simulink model "RM3"  (R2018b)
settings: Solver=ode45  StartTime=0  StopTime=300  FixedStep=0.1  MaxStep=0.1  RelTol=1e-3  EnableMultiTasking=on
values from neighbouring files (symbols this model uses):
  waves = waveClass('regular')    [wecSimInputFile.m]    (also in wecSimInputFileold.m)
undefined symbols (not defined in the file or in its folder): body, constraint, pto, X, Y, Z
libraries: nesl_utility x9, sm_lib x5, WECSim_Lib x4
settings Model: Creator=mlawson  LastModifiedBy=David
settings SolverCC: ZeroCrossControl=DisableAll  AlgebraicLoopSolver=LineSearch  AutoInsertRateTranBlk=on
settings DataIOCC: SaveFormat=Array  SaveOutput=off  SaveTime=off
settings OptimizationCC: LifeSpan=inf  SimCompilerOptimization=on
settings DebuggingCC: UnderspecifiedInitializationDetection=Classic  MergeDetectMultiDrivingBlocksExec=none  SolverPrmCheckMsg=warning  AllowSymbolicDim=off  StateNameClashWarn=warning  SFUnexpectedBacktrackingDiag=warning  SFNoUnconditionalDefaultTransitionDiag=warning  SFExecutionAtInitializationDiag=none
settings HardwareCC: ProdBitPerPointer=32  ProdBitPerSizeT=32  ProdBitPerPtrDiffT=32  ProdLargestAtomicFloat=None  ProdIntDivRoundTo=Undefined  ProdEndianess=Unspecified  ProdWordSize=32  ProdHWDeviceType=32-bit Generic
settings ModelReferenceCC: PropagateSignalLabelsOutOfModel=off
settings SFSimCC: SimUseLocalCustomCode=off
settings RTWCC: RTWUseLocalCustomCode=off
settings CodeAppCC: StateflowObjectComments=on
settings GRTTargetCC: TargetLangStandard=C89/C90 (ANSI)  GeneratePreprocessorConditionals=Disable all
settings ConfigComp: CovMetricSettings=dw  CovHtmlReporting=on  CovSaveCumulativeToWorkspaceVar=on  CovSaveSingleToWorkspaceVar=on  CovExternalEMLEnable=off  CovSFcnEnable=off
settings SimscapeCC: SimscapeNormalizeSystem=off
settings ConfigurationSet: Description=SimMechanics 2G
settings ExplorerConfigSet: InternalSimMechanicsExplorerSettings="<ExplorerConfiguration><canonicalview>default</canonicalview><TilePanel><TileInfo><Tiles Columns=\"1\" Count=\"1\" Rows=\"1\"><Column Left=\"2\" Weight=\"1\"/><Column Left=\"1335\"/><Row Top=\"2\" Weight=\"1\"/><Row Top=\"911\"/><Tile Height=\"1\" Width=\"1\" X=\"0\" Y=\"0\"/></Tiles></TileInfo><SceneInfo><SceneViewer><BGColor><R>0.60000002384185791</R><G>0.60000002384185791</G><B>0.60000002384185791</B></BGColor><Camera><Position><X>365.37645888990272</X><Y>-369.82486814446582</Y><Z>359.64809521743916</Z></Position><Center><X>-6.7351450971904585</X><Y>2.2867358426280204</Y><Z>-12.463508769654169</Z></Center><Up><X>-0.40824829046386307</X><Y>0.40824829046386307</Y><Z>0.81649658092772615</Z></Up><Left>-57.820127362122818</Left><Right>57.820127362122818</Right><Bottom>-38.308817187253304</Bottom><Top>38.308817187253304</Top></Camera></SceneViewer></SceneInfo></TilePanel></ExplorerConfiguration>"

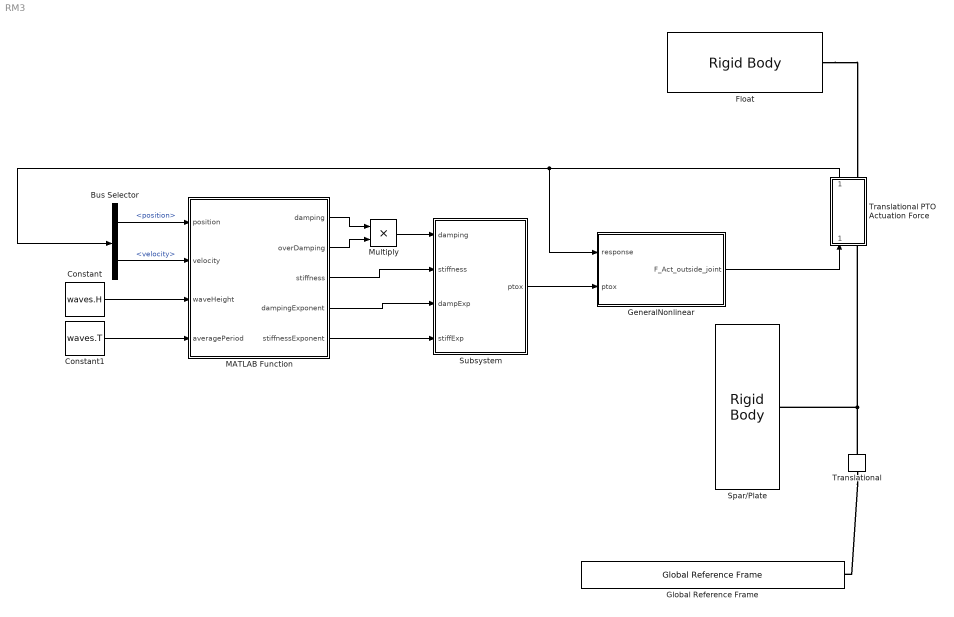
== system RM3 ==
  Bus Selector : BusSelector  OutputSignals=position,velocity
  Constant : Constant  Value=waves.H
  Constant1 : Constant  Value=waves.T
  Float : WECSim_Lib/Body Elements/Rigid Body  body=body(1)
      settings: AttributesFormatString=%<body>  SourceProductName=WEC-Sim
  GeneralNonlinear : Subsystem
  Global Reference Frame : WECSim_Lib/Frames/Global Reference Frame  waves=waves  simu=simu
      settings: SourceProductName=WEC-Sim
  MATLAB Function : MATLAB Function  TreatAsAtomicUnit=on
  Multiply : Product
  Spar/Plate : WECSim_Lib/Body Elements/Rigid Body  body=body(2)
      settings: AttributesFormatString=%<body>  SourceProductName=WEC-Sim
  Subsystem : Subsystem
  Translational : WECSim_Lib/Constraints/Translational  constraint=constraint(1)
      settings: AttributesFormatString=%<constraint>  SourceProductName=WEC-Sim
  Translational PTO Actuation Force : Subsystem  AncestorBlock=WECSim_Lib/PTOs/Translational PTO Actuation Force  mask(PTO){pto=pto(1)}
      mask prompts: pto "PTO Name:"
      mask help:
      | Constraints the follower to translational motion relative to the base, in
      | the PTO's Z-direction and adds PTO stiffness and damping. Also applies a
      | user-defined force and outputs extension, velocity, and acceleration.
      |
      |
      | The variable name input below must be 'pto(i)' where i=1,2,...
      | pto(i) must be defined in the input file with the following fields:
      |
      |     .name (required)
      |             String.
      |             PTO name. Must comply with Matlab's variable naming rules.
      |     .loc (optional)
      |             3x1 vector [x y z] in meters.
      |             PTO location. Default = [0 0 0]
      |     .k (optional)
      |             Float.
      |             PTO linear spring stiffness. Default = 0
      |     .c (optional)
      |             Float.
      |             PTO linear damping coefficient. Default = 0
      |     .orientation.z (optional)
      |             3x1 vector [x y z].
      |             Direction of the PTO's Z-coordinate. Default = [0 0 1]
      |     .orientation.y (optional)
      |             3x1 vector [x y z].
      |             Direction of the PTO's Y-coordinate. Default = [0 1 0]
      mask init:
      | if exist('pto','var')
      |     h=[gcb '/output'];
      |     responseName=['pto' num2str(pto.ptoNum) '_out'];
      |     set_param(h,'VariableName',responseName);
      | end
      | 
      | pto.checkLoc('W');
      settings: AttributesFormatString=%<pto>
      mask Help:
      | Constraints the follower to translational motion relative to the base, in
      | the PTO's Z-direction and adds PTO stiffness and damping. Also applies a
      | user-defined force and outputs extension, velocity, and acceleration.
      | 
      | 
      | The variable name input below must be 'pto(i)' where i=1,2,...
      | pto(i) must be defined in the input file with the following fields:
      | 
      |     .name (required)
      |             String.
      |             PTO name. Must comply with Matlab's variable naming rules.
      |     .loc (optional)
      |             3x1 vector [x y z] in meters.
      |             PTO location. Default = [0 0 0]
      |     .k (optional)
      |             Float.
      |             PTO linear spring stiffness. Default = 0
      |     .c (optional)
      |             Float.
      |             PTO linear damping coefficient. Default = 0
      |     .orientation.z (optional)
      |             3x1 vector [x y z].
      |             Direction of the PTO's Z-coordinate. Default = [0 0 1]
      |     .orientation.y (optional)
      |             3x1 vector [x y z].
      |             Direction of the PTO's Y-coordinate. Default = [0 1 0]
  wires:
  Translational PTO Actuation Force/1(Response) -> Bus Selector/1, GeneralNonlinear/1(response)
  GeneralNonlinear/1(F_Act_outside_joint) -> Translational PTO Actuation Force/1(Force)
  Subsystem/1(ptox) -> GeneralNonlinear/2(ptox)
  Bus Selector/1 -> MATLAB Function/1(position)  "<position>"
  Bus Selector/2 -> MATLAB Function/2(velocity)  "<velocity>"
  Constant/1 -> MATLAB Function/3(waveHeight)
  Constant1/1 -> MATLAB Function/4(averagePeriod)
  MATLAB Function/1(damping) -> Multiply/1
  MATLAB Function/2(overDamping) -> Multiply/2
  MATLAB Function/4(dampingExponent) -> Subsystem/3(dampExp)
  MATLAB Function/5(stiffnessExponent) -> Subsystem/4(stiffExp)
  Multiply/1 -> Subsystem/1(damping)
  MATLAB Function/3(stiffness) -> Subsystem/2(stiffness)
  connections:
  Translational/LConn1 -- Global Reference Frame/RConn1
  Translational/RConn1 -- Translational PTO Actuation Force/LConn1 -- Spar/Plate/RConn1
  Float/RConn1 -- Translational PTO Actuation Force/RConn1

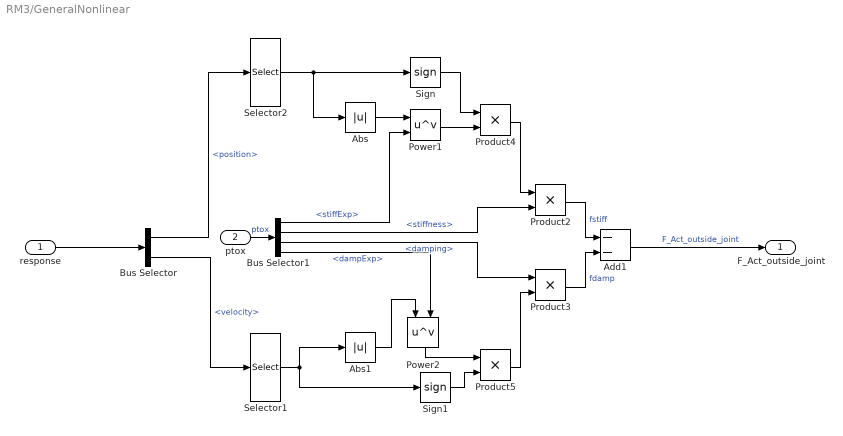
== system RM3/GeneralNonlinear ==
  response : Inport
  ptox : Inport  Port=2
  Abs : Abs
  Abs1 : Abs
  Add1 : Sum  Inputs=--
  Bus Selector : BusSelector  OutputSignals=position,velocity
  Bus Selector1 : BusSelector  OutputSignals=stiffExp,stiffness,damping,dampExp
  Power1 : Math  Operator=pow  SaturateOnIntegerOverflow=on
  Power2 : Math  Operator=pow  SaturateOnIntegerOverflow=on
  Product2 : Product  Inputs=**
  Product3 : Product  Inputs=**
  Product4 : Product
  Product5 : Product
  Selector1 : Selector  InputPortWidth=6  IndexOptions=Index vector (dialog)  Indices=3  OutputSizes=1
  Selector2 : Selector  InputPortWidth=6  IndexOptions=Index vector (dialog)  Indices=3  OutputSizes=1
  Sign : Signum
  Sign1 : Signum
  F_Act_outside_joint : Outport
  wires:
  Power2/1 -> Product5/1
  Product5/1 -> Product3/2
  Sign/1 -> Product4/1
  Bus Selector1/3 -> Product3/1  "<damping>"
  Product2/1 -> Add1/1  "fstiff"
  response/1 -> Bus Selector/1
  Bus Selector1/1 -> Power1/2  "<stiffExp>"
  Bus Selector/2 -> Selector1/1  "<velocity>"
  Selector2/1 -> Sign/1, Abs/1
  Product4/1 -> Product2/1
  Add1/1 -> F_Act_outside_joint/1  "F_Act_outside_joint"
  Abs1/1 -> Power2/1
  Product3/1 -> Add1/2  "fdamp"
  Sign1/1 -> Product5/2
  Bus Selector1/2 -> Product2/2  "<stiffness>"
  Selector1/1 -> Abs1/1, Sign1/1
  Power1/1 -> Product4/2
  Bus Selector/1 -> Selector2/1  "<position>"
  Abs/1 -> Power1/1
  ptox/1 -> Bus Selector1/1  "ptox"
  Bus Selector1/4 -> Power2/2  "<dampExp>"

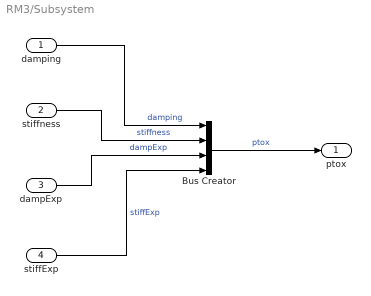
== system RM3/Subsystem ==
  damping : Inport
  stiffness : Inport  Port=2
  dampExp : Inport  Port=3
  stiffExp : Inport  Port=4
  Bus Creator : BusCreator  Inputs=4
  ptox : Outport
  wires:
  stiffness/1 -> Bus Creator/2  "stiffness"
  stiffExp/1 -> Bus Creator/4  "stiffExp"
  Bus Creator/1 -> ptox/1  "ptox"
  damping/1 -> Bus Creator/1  "damping"
  dampExp/1 -> Bus Creator/3  "dampExp"

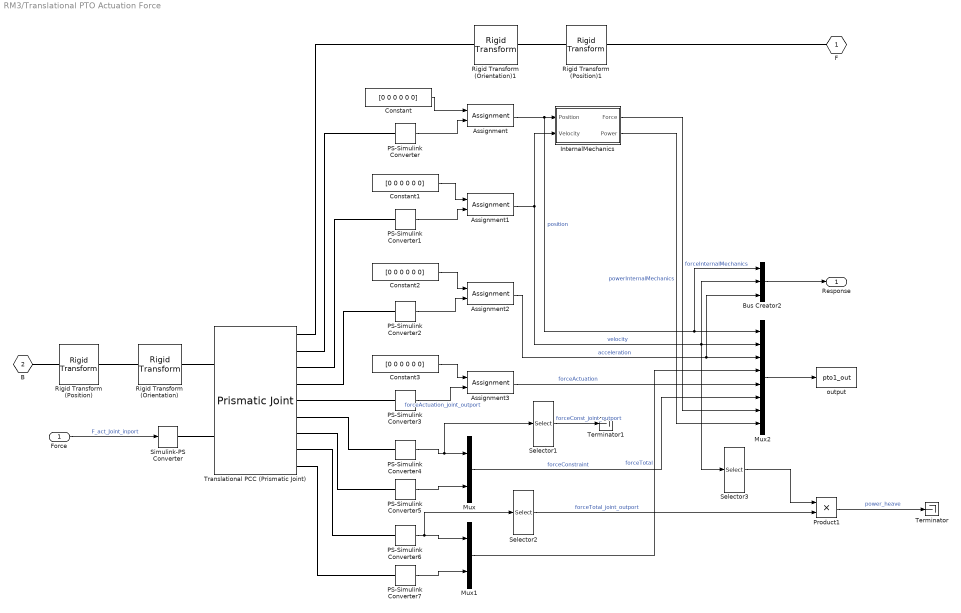
== system RM3/Translational PTO Actuation Force ==
  Force : Inport
  Assignment{,1..3} (4 alike) : Assignment  IndexOptions=Index vector (dialog)  Indices=3  OutputSizes=1
  Bus Creator2 : BusCreator  Inputs=3
  Constant{,1..3} (4 alike) : Constant  Value=[0 0 0 0 0 0]
  InternalMechanics : Subsystem
  Mux : Mux  Inputs=2
  Mux1 : Mux  Inputs=2
  Mux2 : Mux  Inputs=8
  PS-Simulink Converter{,1..7} (8 alike) : nesl_utility/PS-Simulink Converter  PhysicalDomain=network_engine_domain  SubClassName=ps_output  LeftPortType=input  RightPortType=output  PseudoPeriodic=off  Frequencies=[]  Unit=1  AffineConversion=off
  Product1 : Product
  Rigid Transform (Position) : sm_lib/Frames and Transforms/Rigid Transform  TranslationMethod=Cartesian  TranslationStandardOffset=0  TranslationLengthUnit=m  TranslationStandardAxis=+Z  TranslationCartesianOffset=pto.initDisp.initLinDisp + pto.loc  TranslationROffset=0  TranslationROffsetUnits=m  TranslationZOffset=0  TranslationZOffsetUnits=m  TranslationThetaOffset=0  TranslationThetaOffsetUnits=deg  RotationMethod=None  RotationAngleUnits=rad  RotationStandardAxis=+Y  RotationAngle=0  RotationArbitraryAxis=[0 1 0]  FollAlignAxisA=+X  BaseAlignAxisA=+Y  FollAlignAxisB=+Y  BaseAlignAxisB=+Z  RotationSequenceAxes=FollowerAxes  RotationSequence=XYX  RotationSequenceAngles=[0 0 0]  RotationSequenceAnglesUnits=deg  RotationMatrix=[1 0 0; 0 1 0; 0 0 1]
  Rigid Transform (Position)1 : sm_lib/Frames and Transforms/Rigid Transform  TranslationMethod=Cartesian  TranslationStandardOffset=0  TranslationLengthUnit=m  TranslationStandardAxis=+Z  TranslationCartesianOffset=pto.initDisp.initLinDisp + pto.loc  TranslationROffset=0  TranslationROffsetUnits=m  TranslationZOffset=0  TranslationZOffsetUnits=m  TranslationThetaOffset=0  TranslationThetaOffsetUnits=deg  RotationMethod=None  RotationAngleUnits=rad  RotationStandardAxis=+Y  RotationAngle=0  RotationArbitraryAxis=[0 1 0]  FollAlignAxisA=+X  BaseAlignAxisA=+Y  FollAlignAxisB=+Y  BaseAlignAxisB=+Z  RotationSequenceAxes=FollowerAxes  RotationSequence=XYX  RotationSequenceAngles=[0 0 0]  RotationSequenceAnglesUnits=deg  RotationMatrix=[1 0 0; 0 1 0; 0 0 1]
  Rigid Transform (Orientation) : sm_lib/Frames and Transforms/Rigid Transform  TranslationMethod=None  TranslationStandardOffset=0  TranslationLengthUnit=m  TranslationStandardAxis=+Z  TranslationCartesianOffset=0  TranslationROffset=0  TranslationROffsetUnits=m  TranslationZOffset=0  TranslationZOffsetUnits=m  TranslationThetaOffset=0  TranslationThetaOffsetUnits=deg  RotationMethod=RotationMatrix  RotationAngleUnits=rad  RotationStandardAxis=+Y  RotationAngle=0  RotationArbitraryAxis=[0 1 0]  FollAlignAxisA=+X  BaseAlignAxisA=+Y  FollAlignAxisB=+Y  BaseAlignAxisB=+Z  RotationSequenceAxes=FollowerAxes  RotationSequence=XYX  RotationSequenceAngles=[0 0 0]  RotationSequenceAnglesUnits=deg  RotationMatrix=pto.orientation.rotationMatrix
  Rigid Transform (Orientation)1 : sm_lib/Frames and Transforms/Rigid Transform  TranslationMethod=None  TranslationStandardOffset=0  TranslationLengthUnit=m  TranslationStandardAxis=+Z  TranslationCartesianOffset=0  TranslationROffset=0  TranslationROffsetUnits=m  TranslationZOffset=0  TranslationZOffsetUnits=m  TranslationThetaOffset=0  TranslationThetaOffsetUnits=deg  RotationMethod=RotationMatrix  RotationAngleUnits=rad  RotationStandardAxis=+Y  RotationAngle=0  RotationArbitraryAxis=[0 1 0]  FollAlignAxisA=+X  BaseAlignAxisA=+Y  FollAlignAxisB=+Y  BaseAlignAxisB=+Z  RotationSequenceAxes=FollowerAxes  RotationSequence=XYX  RotationSequenceAngles=[0 0 0]  RotationSequenceAnglesUnits=deg  RotationMatrix=pto.orientation.rotationMatrix
  Selector1 : Selector  InputPortWidth=3  IndexOptions=Index vector (dialog)  Indices=3  OutputSizes=1
  Selector2 : Selector  InputPortWidth=3  IndexOptions=Index vector (dialog)  Indices=3  OutputSizes=1
  Selector3 : Selector  InputPortWidth=6  IndexOptions=Index vector (dialog)  Indices=3  OutputSizes=1
  Simulink-PS Converter : nesl_utility/Simulink-PS Converter  PhysicalDomain=network_engine_domain  SubClassName=ps_input  LeftPortType=input  RightPortType=output  PseudoPeriodic=off  Frequencies=[]  NoiseDistribution=none  NoiseParameters=[]  Unit=1  AffineConversion=off  FilteringAndDerivatives=zero  SimscapeFilterOrder=1  InputFilterTimeConstant=0.001  UdotUserProvided=1
  Terminator : Terminator
  Terminator1 : Terminator
  Translational PCC (Prismatic Joint) : sm_lib/Joints/Prismatic Joint  SenseConstraintForce=on  SenseConstraintForceX=off  SenseConstraintForceY=off  SenseConstraintForceZ=off  SenseConstraintTorque=on  SenseConstraintTorqueX=off  SenseConstraintTorqueY=off  SenseConstraintTorqueZ=off  SenseTotalForce=on  SenseTotalForceX=off  SenseTotalForceY=off  SenseTotalForceZ=off  SenseTotalTorque=on  SenseTotalTorqueX=off  SenseTotalTorqueY=off  SenseTotalTorqueZ=off  CompositeWrenchDir=BaseOnFollower  CompositeWrenchFrame=BaseFrame  EquilibriumPosition=0  EquilibriumPositionUnits=m  SpringStiffness=pto.k  SpringStiffnessUnits=N/m  DampingCoefficient=pto.c  DampingCoefficientUnits=N/(m/s)  TorqueActuationMode=InputTorque  MotionActuationMode=ComputedMotion  SensePosition=on  SenseVelocity=on  SenseAcceleration=on  SenseTorqueForce=on  PositionTargetSpecify=off  PositionTargetPriority=High  PositionTargetValue=0  PositionTargetValueUnits=m  VelocityTargetSpecify=off  VelocityTargetPriority=High  VelocityTargetValue=0  VelocityTargetValueUnits=m/s
  output : ToWorkspace  VariableName=pto1_out  SaveFormat=Structure With Time  SampleTime=-1
      settings: Decimation=round(simu.dtOut/simu.dt,0)
  F : PMIOPort  Side=Right
  B : PMIOPort  Port=2  Side=Left
  Response : Outport
  wires:
  Bus Creator2/1 -> Response/1
  Assignment/1 -> Mux2/1, Bus Creator2/1, InternalMechanics/1(Position)  "position"
  Assignment1/1 -> Selector3/1, Bus Creator2/2, Mux2/2, InternalMechanics/2(Velocity)  "velocity"
  Assignment2/1 -> Mux2/3, Bus Creator2/3  "acceleration"
  Force/1 -> Simulink-PS Converter/1  "F_act_Joint_inport"
  Mux2/1 -> output/1
  Mux/1 -> Mux2/6  "forceConstraint"
  Mux1/1 -> Mux2/4  "forceTotal"
  PS-Simulink Converter5/1 -> Mux/2
  PS-Simulink Converter6/1 -> Selector2/1, Mux1/1
  PS-Simulink Converter7/1 -> Mux1/2
  Assignment3/1 -> Mux2/5  "forceActuation"
  Constant/1 -> Assignment/1
  PS-Simulink Converter/1 -> Assignment/2
  Constant1/1 -> Assignment1/1
  PS-Simulink Converter1/1 -> Assignment1/2
  Constant2/1 -> Assignment2/1
  PS-Simulink Converter2/1 -> Assignment2/2
  InternalMechanics/1(Force) -> Mux2/7  "forceInternalMechanics"
  InternalMechanics/2(Power) -> Mux2/8  "powerInternalMechanics"
  Constant3/1 -> Assignment3/1
  PS-Simulink Converter3/1 -> Assignment3/2  "forceActuation_joint_outport"
  Selector2/1 -> Product1/2  "forceTotal_joint_outport"
  PS-Simulink Converter4/1 -> Selector1/1, Mux/1
  Selector1/1 -> Terminator1/1  "forceConst_joint_outport"
  Product1/1 -> Terminator/1  "power_heave"
  Selector3/1 -> Product1/1
  connections:
  Rigid Transform (Position)/RConn1 -- Rigid Transform (Orientation)/LConn1
  Rigid Transform (Position)1/RConn1 -- Rigid Transform (Orientation)1/LConn1
  Simulink-PS Converter/RConn1 -- Translational PCC (Prismatic Joint)/LConn2
  Rigid Transform (Orientation)/RConn1 -- Translational PCC (Prismatic Joint)/LConn1
  Rigid Transform (Position)/LConn1 -- B/RConn1
  Translational PCC (Prismatic Joint)/RConn5 -- PS-Simulink Converter3/LConn1
  Translational PCC (Prismatic Joint)/RConn9 -- PS-Simulink Converter7/LConn1
  Rigid Transform (Orientation)1/RConn1 -- Translational PCC (Prismatic Joint)/RConn1
  Translational PCC (Prismatic Joint)/RConn4 -- PS-Simulink Converter2/LConn1
  Translational PCC (Prismatic Joint)/RConn7 -- PS-Simulink Converter5/LConn1
  Translational PCC (Prismatic Joint)/RConn3 -- PS-Simulink Converter1/LConn1
  Rigid Transform (Position)1/LConn1 -- F/RConn1
  Translational PCC (Prismatic Joint)/RConn8 -- PS-Simulink Converter6/LConn1
  Translational PCC (Prismatic Joint)/RConn2 -- PS-Simulink Converter/LConn1
  Translational PCC (Prismatic Joint)/RConn6 -- PS-Simulink Converter4/LConn1

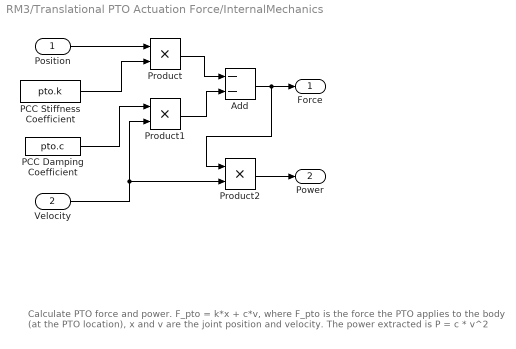
== system RM3/Translational PTO Actuation Force/InternalMechanics ==
  note: Calculate PTO force and power.
      |
      | F_pto  = k*x + c*v,
      | where F_pto is the force the PTO applies to the body (at the PTO location), x and v are the joint position and velocity.
      |
      | The power extracted is
      | P = c * v^2
  Position : Inport
  Velocity : Inport  Port=2
  Add : Sum  Inputs=--
  PCC Damping Coefficient : Constant  Value=pto.c
  PCC Stiffness Coefficient : Constant  Value=pto.k
  Product : Product  Inputs=**
  Product1 : Product  Inputs=**
  Product2 : Product  Inputs=**
  Force : Outport
  Power : Outport  Port=2
  wires:
  PCC Damping Coefficient/1 -> Product1/1
  Product2/1 -> Power/1
  PCC Stiffness Coefficient/1 -> Product/2
  Position/1 -> Product/1
  Add/1 -> Product2/1, Force/1
  Velocity/1 -> Product1/2, Product2/2
  Product/1 -> Add/1
  Product1/1 -> Add/2

== matlab function RM3/MATLAB Function ==
  data: position input; velocity input; waveHeight input; damping output; overDamping output; averagePeriod input; stiffness output; dampingExponent output; stiffnessExponent output
function [damping, overDamping, stiffness, dampingExponent, stiffnessExponent] =...
    fuzzyLogicController(position, velocity, waveHeight, averagePeriod)


start = tic;
verbose = 1;


%%%%%%%%%%%%%%%%%%%%%%%%%%%%%%%%%%%%%%%
%% Define input membership functions %%
%%%%%%%%%%%%%%%%%%%%%%%%%%%%%%%%%%%%%%%

%%% Waveheight Input %%%

    % Low waveheight open trap MF
    fS.inputs.waveHeight.MFs.low.type = 'down step';
    fS.inputs.waveHeight.MFs.low.begin = 0.41;
    fS.inputs.waveHeight.MFs.low.finish = 1.40;

    % Medium Low (Q1) waveheight triangular MF
    fS.inputs.waveHeight.MFs.medLow.type = 'triangle';
    fS.inputs.waveHeight.MFs.medLow.begin = 0.41;
    fS.inputs.waveHeight.MFs.medLow.peak = 1.40;
    fS.inputs.waveHeight.MFs.medLow.finish = 1.88;

    % Medium (median) waveheight triangular MF
    fS.inputs.waveHeight.MFs.med.type = 'triangle';
    fS.inputs.waveHeight.MFs.med.begin = 1.40;
    fS.inputs.waveHeight.MFs.med.peak = 1.88;
    fS.inputs.waveHeight.MFs.med.finish = 2.65;

    % Medium High (Q3) waveheight triangular MF
    fS.inputs.waveHeight.MFs.medHigh.type = 'triangle';
    fS.inputs.waveHeight.MFs.medHigh.begin = 1.88;
    fS.inputs.waveHeight.MFs.medHigh.peak = 2.65;
    fS.inputs.waveHeight.MFs.medHigh.finish = 10.43;

    % High waveheight open trap MF
    fS.inputs.waveHeight.MFs.high.type = 'step';
    fS.inputs.waveHeight.MFs.high.begin = 2.65;
    fS.inputs.waveHeight.MFs.high.finish = 10.43; 

%%% Average Wave Period Input %%%

    % Low period open trap MF
    fS.inputs.avgPeriod.MFs.short.type = 'down step';
    fS.inputs.avgPeriod.MFs.short.begin = 3.52;
    fS.inputs.avgPeriod.MFs.short.finish = 5.94;

    % Medium Low (Q1) period triangular MF
    fS.inputs.avgPeriod.MFs.midShort.type = 'triangle';
    fS.inputs.avgPeriod.MFs.midShort.begin = 3.52;
    fS.inputs.avgPeriod.MFs.midShort.peak = 5.94;
    fS.inputs.avgPeriod.MFs.midShort.finish = 6.81;

    % Medium (median) period triangular MF
    fS.inputs.avgPeriod.MFs.mid.type = 'triangle';
    fS.inputs.avgPeriod.MFs.mid.begin = 5.94;
    fS.inputs.avgPeriod.MFs.mid.peak = 6.81;
    fS.inputs.avgPeriod.MFs.mid.finish = 7.89;

    % Medium High (Q3) period triangular MF
    fS.inputs.avgPeriod.MFs.midLong.type = 'triangle';
    fS.inputs.avgPeriod.MFs.midLong.begin = 6.81;
    fS.inputs.avgPeriod.MFs.midLong.peak = 7.89;
    fS.inputs.avgPeriod.MFs.midLong.finish = 12.97;

    % High period open trap MF
    fS.inputs.avgPeriod.MFs.long.type = 'step';
    fS.inputs.avgPeriod.MFs.long.begin = 7.89;
    fS.inputs.avgPeriod.MFs.long.finish = 12.97;

%%% Velocity Input %%%

    % Too fast Negative Velocity Limit
    fS.inputs.velocity.MFs.fastNeg.type = 'down step';
    fS.inputs.velocity.MFs.fastNeg.begin = -1;
    fS.inputs.velocity.MFs.fastNeg.finish = 0;
    
    % In spec speeds
    fS.inputs.velocity.MFs.slow.type = 'triangle';
    fS.inputs.velocity.MFs.slow.begin = -1;
    fS.inputs.velocity.MFs.slow.peak = 0;
    fS.inputs.velocity.MFs.slow.finish = 1;
    
    % Too Fast Positive Velocity
    fS.inputs.velocity.MFs.fastPos.type = 'step';
    fS.inputs.velocity.MFs.fastPos.begin = 0;
    fS.inputs.velocity.MFs.fastPos.finish = 1;

%%% Position Input %%%

    % Too Negative Position Limit
    fS.inputs.position.MFs.low.type = 'down step';
    fS.inputs.position.MFs.low.begin = -1;
    fS.inputs.position.MFs.low.finish = -0.75;
    
    % In spec speeds
    fS.inputs.position.MFs.middle.type = 'trap';
    fS.inputs.position.MFs.middle.begin = -1;
    fS.inputs.position.MFs.middle.asc = -0.75;
    fS.inputs.position.MFs.middle.dec = 0.75;
    fS.inputs.position.MFs.middle.finish = 1;
    
    % Too Positive Position
    fS.inputs.position.MFs.high.type = 'step';
    fS.inputs.position.MFs.high.begin = 0.75;
    fS.inputs.position.MFs.high.finish = 1;

%%%%%%%%%%%%%%%%%%
%% Define Rules %%
%%%%%%%%%%%%%%%%%%
% Define Rules for outputs, Define Fuzzy Operators, (for speed and position, 
% any rule with multiple inputs), define each rule's implication method,
% define aggregation method for determining outputs for all rules 





%%%%%%%%%%%%%%%%%%
%% Fuzzify Inputs %%
%%%%%%%%%%%%%%%%%%
fS.inputs.waveHeight.MFs = evaluate_MFs(waveHeight, fS.inputs.waveHeight.MFs);
fS.inputs.avgPeriod.MFs = evaluate_MFs(averagePeriod, fS.inputs.avgPeriod.MFs);
fS.inputs.position.MFs = evaluate_MFs(position, fS.inputs.position.MFs);
fS.inputs.velocity.MFs = evaluate_MFs(velocity, fS.inputs.velocity.MFs);

if verbose % print firings
    listInputs = fieldnames(fS.inputs);
    for i=1:numel(listInputs)
        firings = [];
        thisInput = fS.inputs.(listInputs{i});
        disp(listInputs{i});
        listMFs = fieldnames(fS.inputs.(listInputs{i}).MFs);
        for k=1:numel(listMFs)
             thisMF = fS.inputs.(listInputs{i}).MFs.(listMFs{k});
             firings = [firings thisMF.firing];
        end
        disp('firings');
        disp(firings);
    end
end

%% Apply Fuzzy Operator %%

%% Apply Implication for rules %%

%% Aggregation outputs for all rules %%


[damping, overDamping, stiffness, dampingExponent, stiffnessExponent] =


%%%%%%%%%%%%%%%%%%
%% End of Main %%
%%%%%%%%%%%%%%%%%%
% begin functions

function Evaluated_MFs = evaluate_MFs(inValue, MFs)

    % list of memberships for this input
    listMFs = fieldnames(MFs);

    % go through each membership and 
    for k=1:numel(listMFs)
        thisMF = MFs.(listMFs{k});

        MF_Type = thisMF.type;

        %calculate its firing strength based on
        switch MF_Type
            case 'triangle'
                % TODO: sanitize inputs (if not start -> peak -> finish)
                MFs.(listMFs{k}).firing = tri_MF(inValue,...
                    thisMF.begin, thisMF.peak, thisMF.finish);
            case 'step'
                MFs.(listMFs{k}).firing = open_trap_right(inValue,...
                     thisMF.begin, thisMF.finish);
            case 'down step'
                 %sanitize inputs (if not start -> peak -> finish)
                 MFs.(listMFs{k}).firing = open_trap_left(inValue,...
                     thisMF.begin, thisMF.finish);
            case 'trap'
                 %sanitize inputs (if not start -> peak -> finish)
                 MFs.(listMFs{k}).firing = trap(inValue,...
                     thisMF.begin, thisMF.asc, thisMF.dec, thisMF.finish);
        end

    end

    Evaluated_MFs = MFs;

end

function membership = tri_MF(inValue, begin, peak, finish)

% Evaluate input according to triangular input MF
if inValue <= peak
    if inValue < begin
        membership = 0;
    else
        membership = (1/(peak - begin)) * (inValue-peak) + 1;
    end
elseif inValue > peak
    if inValue > finish
        membership = 0;
    else
        membership = (-1/(finish - peak)) * (inValue-peak) + 1;
    end
else
    membership = 1;
end

end

function membership = open_trap_left(inValue, begin, finish)

if inValue < begin
     membership = 1;
 elseif inValue > finish
     membership = 0;
 else
     membership = (1/(begin - finish))*(inValue - begin) + 1;
end

end

function membership = open_trap_right(inValue, begin, finish)
 if inValue < begin
     membership = 0;
 elseif inValue > finish
     membership = 1;
 else
     membership = (1/(finish - begin))*(inValue - finish) + 1;
 end
end


function membership = trap(inValue, begin, asc, dec, finish)
 if ( inValue < begin ) || ( inValue > finish )
     membership = 0;
 elseif inValue < asc
     membership = (1/(asc-begin))*(inValue - begin);
 elseif inValue > dec
     membership = (1/(dec-finish))*(inValue - finish);
 else
     membership = 1;
 end
end

end
